simulink model "odev1_22"  (R2019b)
settings: Solver=VariableStepAuto  StartTime=0.0  StopTime=50  RelTol=1e-3
settings Model: Creator=Mustafa Sezer  LastModifiedBy=Mustafa Sezer

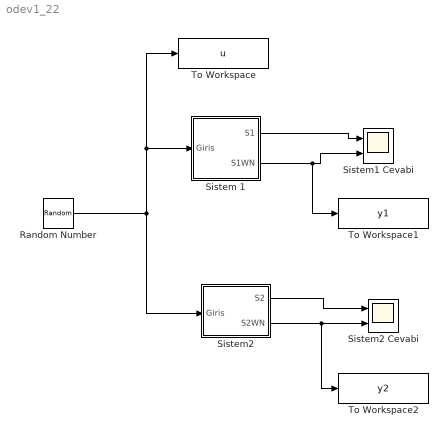
== system odev1_22 ==
  Random Number : RandomNumber  Seed=1  SampleTime=0.1
  Sistem 1 : Subsystem
  Sistem1 Cevabi : Scope  NumInputPorts=2
  Sistem2 : Subsystem
  Sistem2 Cevabi : Scope  NumInputPorts=2
  To Workspace : ToWorkspace  VariableName=u  SaveFormat=Timeseries  SampleTime=-1
  To Workspace1 : ToWorkspace  VariableName=y1  SaveFormat=Timeseries  SampleTime=-1
  To Workspace2 : ToWorkspace  VariableName=y2  SaveFormat=Timeseries  SampleTime=-1
  wires:
  Random Number/1 -> Sistem 1/1(Giris), To Workspace/1, Sistem2/1(Giris)
  Sistem 1/1(S1) -> Sistem1 Cevabi/1
  Sistem2/1(S2) -> Sistem2 Cevabi/1
  Sistem 1/2(S1WN) -> To Workspace1/1, Sistem1 Cevabi/2
  Sistem2/2(S2WN) -> To Workspace2/1, Sistem2 Cevabi/2

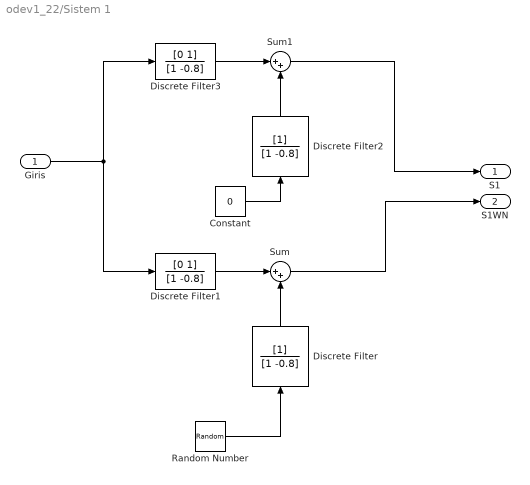
== system odev1_22/Sistem 1 ==
  Giris : Inport
  Constant : Constant  Value=0
  Discrete Filter : DiscreteFilter  Denominator=[1 -0.8]
  Discrete Filter1 : DiscreteFilter  Numerator=[0 1]  Denominator=[1 -0.8]
  Discrete Filter2 : DiscreteFilter  Denominator=[1 -0.8]
  Discrete Filter3 : DiscreteFilter  Numerator=[0 1]  Denominator=[1 -0.8]
  Random Number : RandomNumber  SampleTime=0.1
  Sum : Sum  Inputs=|++
  Sum1 : Sum  Inputs=|++
  S1 : Outport
  S1WN : Outport  Port=2
  wires:
  Discrete Filter/1 -> Sum/2
  Random Number/1 -> Discrete Filter/1
  Discrete Filter3/1 -> Sum1/1
  Constant/1 -> Discrete Filter2/1
  Discrete Filter1/1 -> Sum/1
  Sum/1 -> S1WN/1
  Discrete Filter2/1 -> Sum1/2
  Sum1/1 -> S1/1
  Giris/1 -> Discrete Filter1/1, Discrete Filter3/1

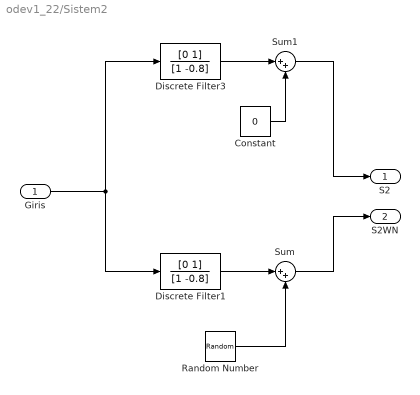
== system odev1_22/Sistem2 ==
  Giris : Inport
  Constant : Constant  Value=0
  Discrete Filter1 : DiscreteFilter  Numerator=[0 1]  Denominator=[1 -0.8]
  Discrete Filter3 : DiscreteFilter  Numerator=[0 1]  Denominator=[1 -0.8]
  Random Number : RandomNumber  SampleTime=0.1
  Sum : Sum  Inputs=|++
  Sum1 : Sum  Inputs=|++
  S2 : Outport
  S2WN : Outport  Port=2
  wires:
  Sum1/1 -> S2/1
  Constant/1 -> Sum1/2
  Random Number/1 -> Sum/2
  Sum/1 -> S2WN/1
  Discrete Filter1/1 -> Sum/1
  Discrete Filter3/1 -> Sum1/1
  Giris/1 -> Discrete Filter1/1, Discrete Filter3/1
